simulink model "velocity_sin"  (R2015b)
settings: Solver=FixedStepDiscrete  StartTime=0.0  StopTime=inf  RelTol=1e-3
undefined symbols (not defined in the file or in its folder): DiscIntNeverNeededParam, Down, GPTRIP1SEL, GPTRIP2SEL, PWM_Counter_Period, TZ1, TZ2, Up
libraries: c280xlib x3, simulink x3, c2806xlib x2, dspsigops x2, c2802xlib x1
settings Model: ExtModeTrigDuration=10  Creator=Kalman  LastModifiedBy=ata.otaran
settings DataIOCC: SaveFormat=Array
settings OptimizationCC: OptimizeModelRefInitCode=on  LifeSpan=Inf  MaxStackSize=512
settings HardwareCC: ProdBitPerChar=16  ProdBitPerInt=16  ProdBitPerPointer=16  ProdLargestAtomicInteger=Integer  ProdLargestAtomicFloat=None  ProdWordSize=16  ProdLongLongMode=on  ProdHWDeviceType=Texas Instruments->C2000
settings RTWCC: SystemTargetFile=ert.tlc  TemplateMakefile=ert_default_tmf  Description=Embedded Coder  Toolchain=Texas Instruments Code Composer Studio v5 (C2000)
settings CodeAppCC: IgnoreCustomStorageClasses=off
settings ERTTargetCC: CodeReplacementLibrary=TI C28x
settings ConfigComp: CovModelRefEnable=Off

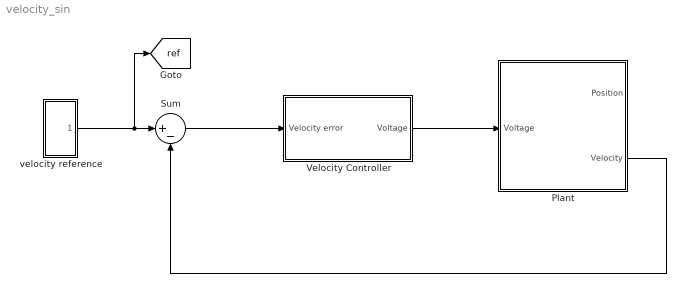
== system velocity_sin ==
  Plant : Subsystem
  Sum : Sum  Inputs=|+-
  Velocity Controller : Subsystem
  velocity reference : Subsystem
  tag scope: ref=global
  wires:
  Sum/1 -> Velocity Controller/1("Velocity error ")
  velocity reference/1(vref) -> [ref], Sum/1
  Plant/2(Velocity) -> Sum/2
  Velocity Controller/1(Voltage) -> Plant/1(Voltage)

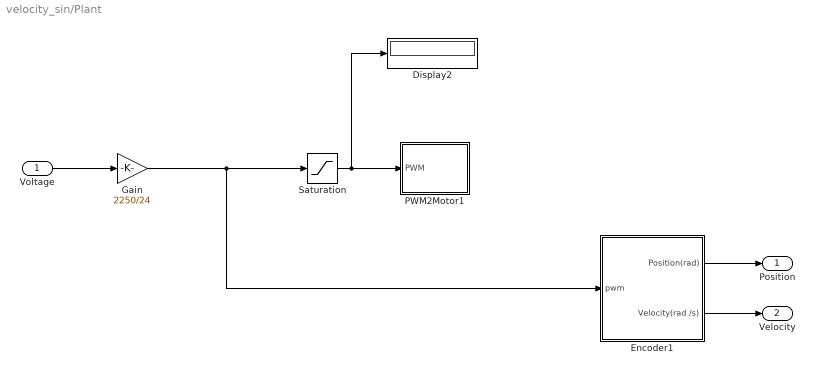
== system velocity_sin/Plant ==
  Voltage : Inport
  Display2 : Display
  Encoder1 : Subsystem
  Gain : Gain  Gain=2250/24
  PWM2Motor1 : Subsystem
  Saturation : Saturate  UpperLimit=2250  LowerLimit=-2250
  Position : Outport
  Velocity : Outport  Port=2
  wires:
  Encoder1/1("Position(rad) ") -> Position/1
  Encoder1/2(Velocity(rad /s)) -> Velocity/1
  Saturation/1 -> PWM2Motor1/1(PWM), Display2/1
  Gain/1 -> Saturation/1, Encoder1/1(pwm)
  Voltage/1 -> Gain/1

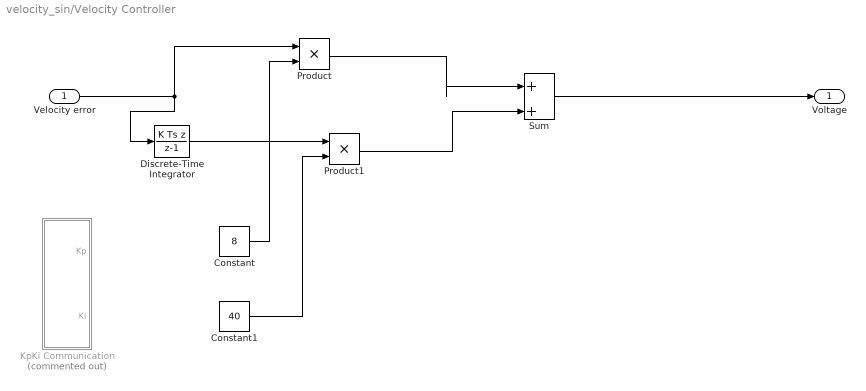
== system velocity_sin/Velocity Controller ==
  "Velocity error " : Inport
  Constant : Constant  Value=8
  Constant1 : Constant  Value=40
  Discrete-Time Integrator : DiscreteIntegrator  IntegratorMethod=Integration: Backward Euler  InitialConditionSetting=State (most efficient)  SampleTime=-1  ICPrevOutput=DiscIntNeverNeededParam  ICPrevScaledInput=DiscIntNeverNeededParam
  KpKi Communication : Subsystem  Commented=on
  Product : Product
  Product1 : Product
  Sum : Sum  Inputs=|++
  Voltage : Outport
  wires:
  "Velocity error "/1 -> Product/1, Discrete-Time Integrator/1
  Product/1 -> Sum/1
  Product1/1 -> Sum/2
  Discrete-Time Integrator/1 -> Product1/1
  Sum/1 -> Voltage/1
  Constant/1 -> Product/2
  Constant1/1 -> Product1/2

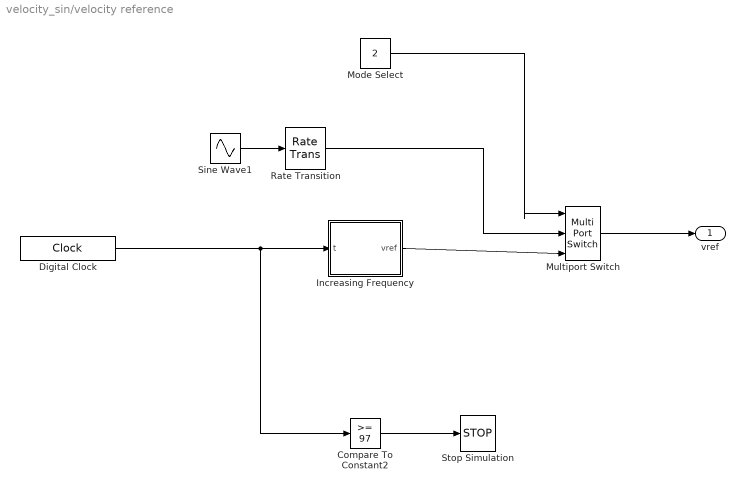
== system velocity_sin/velocity reference ==
  Compare To Constant2 : simulink/Logic and Bit Operations/Compare To Constant  relop=>=  const=97  OutDataTypeStr=boolean
  Digital Clock : DigitalClock  SampleTime=0.0001
  Increasing Frequency : Subsystem
  Mode Select : Constant  Value=2
  Multiport Switch : MultiPortSwitch  Inputs=2
  Rate Transition : RateTransition
  Sine Wave1 : Sin  Amplitude=5  Frequency=2*pi
  Stop Simulation : Stop
  vref : Outport
  wires:
  Sine Wave1/1 -> Rate Transition/1
  Digital Clock/1 -> Compare To Constant2/1, Increasing Frequency/1(t)
  Compare To Constant2/1 -> Stop Simulation/1
  Increasing Frequency/1(vref) -> Multiport Switch/3
  Rate Transition/1 -> Multiport Switch/2
  Multiport Switch/1 -> vref/1
  Mode Select/1 -> Multiport Switch/1

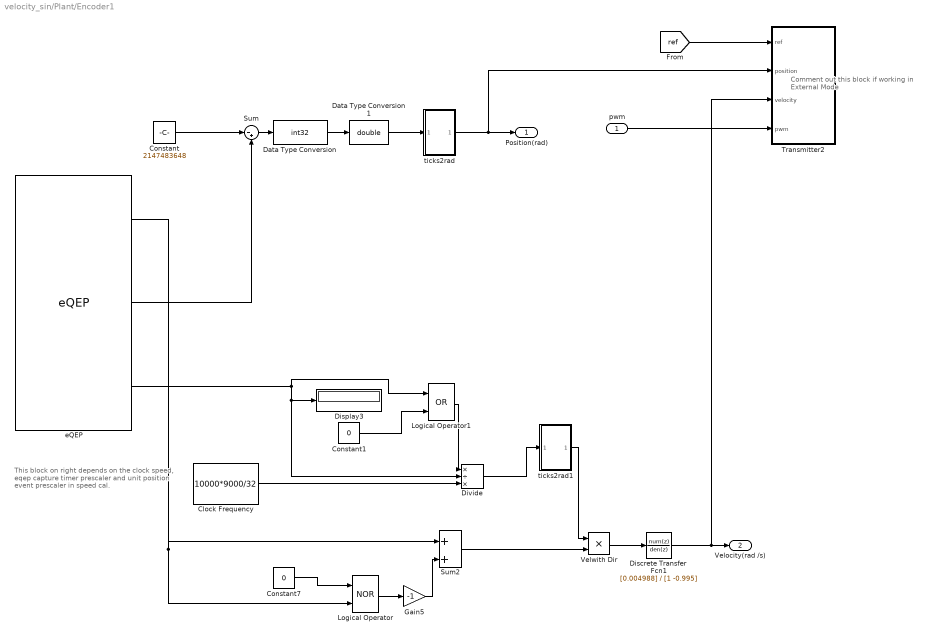
== system velocity_sin/Plant/Encoder1 ==
  note: Comment out this block if
      | working in External Mode
  note: This block on right depends on the clock speed, eqep capture timer prescaler and
      | unit position event prescaler in speed cal.
  pwm : Inport
  Clock Frequency : Constant  Value=10000*9000/32
  Constant : Constant  Value=2147483648  OutDataTypeStr=uint32
  Constant1 : Constant  Value=0
  Constant7 : Constant  Value=0
  Data Type Conversion : DataTypeConversion  OutDataTypeStr=int32
  Data Type Conversion1 : DataTypeConversion  OutDataTypeStr=double
  Discrete Transfer Fcn1 : DiscreteTransferFcn  Numerator=[0.004988]  Denominator=[1 -0.995]
  Display3 : Display
  Divide : Product  Inputs=*/*
  Gain5 : Gain  Gain=-1
  Logical Operator : Logic  Operator=NOR  AllPortsSameDT=off  OutDataTypeStr=boolean
  Logical Operator1 : Logic  Operator=OR  AllPortsSameDT=off  OutDataTypeStr=boolean
  Sum : Sum  Inputs=|-+
  Sum2 : Sum  Inputs=|++
  Transmitter2 : Subsystem
  "Velwith Dir " : Product
  eQEP : c280xlib/eQEP  useModule=eQEP1  pcInputmode=Quadrature-count  externalClockrate=2x resolution: Count the rising/falling edge  swapPolarityselection=Clockwise  qdfOutputport=on  qapPolarityselection=off  qbpPolarityselection=off  qipPolarityselection=off  qspPolarityselection=off  igatePolarityselection=off  sampleTime=0.0001  pcOutputport=on  pcMaximumvalue=4294967295  indexInitializationcheck=off  indexInitializationevent=Rising edge  strobeInitializationcheck=off  strobeInitializationevent=Rising edge  softwareInitializationcheck=on  softwareInitializationsource=Set to init value at start up  softwareInitializationmode=on  pcInitialvalue=2147483648  pcResetmode=Reset on an index event  ieloutputport=off  indexEventlatch=Rising edge  seloutputport=off  strobeEventlatch=Rising edge  pcefOutputport=off  enableEqepcapture=on  qctmrOutputport=off  qcprdOutputport=on  captureTimerprescaler=128  upEventprescaler=4  overflowErrorflag=off  directionErrorflag=off  captureTimerposition=On position counter read  unitTimerperiod=1000000000  captureTimerlatch=off  capturePeriodlatch=off  positionCounterlatch=off  soenPolarityselection=off  spselPolarityselection=Index pin is used for sync output  compareValuesource=Specify via dialog  shadowMode=Load on QPOSCNT=0  compareValue=4294967295  syncOutputwidth=1  polaritySyncoutput=Active high  watchdogEnable=off  watchdogTimer=65535  outport1Datatype=auto  outport2Datatype=uint32  outport3Datatype=auto  outport4Datatype=auto  outport5Datatype=auto  outport6Datatype=auto  outport7Datatype=auto  outport8Datatype=auto  outport9Datatype=auto  outport10Datatype=auto  outport11Datatype=auto  outport12Datatype=auto  eqepinterrupt_pce=off  eqepinterrupt_qpe=off  eqepinterrupt_qdc=off  eqepinterrupt_wto=off  eqepinterrupt_pcu=off  eqepinterrupt_pco=off  eqepinterrupt_pcr=off  eqepinterrupt_pcm=off  eqepinterrupt_sel=off  eqepinterrupt_iel=off  eqepinterrupt_uto=off  pheOutputport=off  watchdogOutputport=off  outport13Datatype=auto  outport14Datatype=auto
  ticks2rad : Subsystem
  ticks2rad1 : Subsystem
  "Position(rad) " : Outport
  Velocity(rad /s) : Outport  Port=2
  wires:
  ticks2rad1/1(Out1) -> "Velwith Dir "/1
  Logical Operator1/1 -> Divide/1
  Clock Frequency/1 -> Divide/3
  Constant1/1 -> Logical Operator1/2
  Sum2/1 -> "Velwith Dir "/2
  Constant7/1 -> Logical Operator/1
  Logical Operator/1 -> Gain5/1
  Divide/1 -> ticks2rad1/1(In1)
  Gain5/1 -> Sum2/2
  eQEP/1 -> Logical Operator/2, Sum2/1
  eQEP/2 -> Sum/2
  Constant/1 -> Sum/1
  eQEP/3 -> Divide/2, Display3/1, Logical Operator1/1
  Data Type Conversion/1 -> Data Type Conversion1/1
  ticks2rad/1(Out1) -> Transmitter2/2(position), "Position(rad) "/1
  Sum/1 -> Data Type Conversion/1
  Data Type Conversion1/1 -> ticks2rad/1(In1)
  pwm/1 -> Transmitter2/4(pwm)
  "Velwith Dir "/1 -> Discrete Transfer Fcn1/1
  [ref] -> Transmitter2/1(ref)
  Discrete Transfer Fcn1/1 -> Transmitter2/3(velocity), Velocity(rad /s)/1

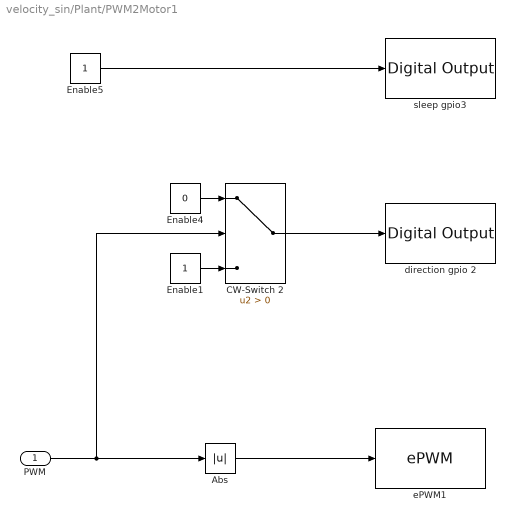
== system velocity_sin/Plant/PWM2Motor1 ==
  PWM : Inport
  Abs : Abs
  CW-Switch 2 : Switch  Criteria=u2 > Threshold
  Enable1 : Constant
  Enable4 : Constant  Value=0
  Enable5 : Constant
  direction gpio 2 : c2806xlib/Digital Output  GPIO_Number=GPIO0~GPIO7  GPIO_Bit0=off  GPIO_BIT0_Toggle=off  GPIO_Bit1=off  GPIO_BIT1_Toggle=off  GPIO_Bit2=on  GPIO_BIT2_Toggle=off  GPIO_Bit3=off  GPIO_BIT3_Toggle=off  GPIO_Bit4=off  GPIO_BIT4_Toggle=off  GPIO_Bit5=off  GPIO_BIT5_Toggle=off  GPIO_Bit6=off  GPIO_BIT6_Toggle=off  GPIO_Bit7=off  GPIO_BIT7_Toggle=off
  ePWM1 : c2802xlib/ePWM  useModule=ePWM1  ePWMxLINKTBPRD=Not Linked  periodUnits=Clock cycles  timerSource=Specify via dialog  timerPeriod_clk=PWM_Counter_Period+1  timerPeriod_sec=0.0001  tbshadow=Counter equals to zero  countingMode=Up-Down  phaseActiveEnable=Disable  phaseDirection=Count down after sync  phaseActive=0  synchronizationEnable=off  dcaevt1Sync=off  dcbevt1Sync=off  synchronizationOption=Disable  clockPrescale=1  HSclockPrescale=1  enswap=off  ePWMxAStatus=on  ePWMxAactionLogic1=Do nothing  ePWMxAactionLogic2=Do nothing  ePWMxAactionLogic3=Clear  ePWMxAactionLogic4=Set  ePWMxAactionLogic5=Do nothing  ePWMxAactionLogic6=Do nothing  ePWMxALoadMode=Load on counter equals to zero (CTR=Zero)  ePWMxACSFenable=off  ePWMxACSFvalue=Forcing disable  ePWMxASFreload=Zero  ePWMxBStatus=off  ePWMxBactionLogic1=Set  ePWMxBactionLogic2=Clear  ePWMxBactionLogic3=Do nothing  ePWMxBactionLogic4=Do nothing  ePWMxBactionLogic5=Clear  ePWMxBactionLogic6=Set  ePWMxBLoadMode=Load on counter equals to zero (CTR=Zero)  ePWMxBCSFenable=off  ePWMxBCSFvalue=Forcing disable  ePWMxBSFreload=Zero  ePWNxBOutWay=off  ePWMxLINKCMPA=Not Linked  CMPAUnits=Clock cycles  CMPASource=Input port  CMPAValue_per=50  CMPAValue_clk=PWM_Counter_Period/2+1  enCMPAshadow=Counter equals to zero  ePWMxLINKCMPB=Not Linked  CMPBUnits=Clock cycles  CMPBSource=Specify via dialog  CMPBValue_per=50  CMPBValue_clk=PWM_Counter_Period/2+1  enCMPBshadow=Counter equals to zero  ePWMxLINKCMPC=Not Linked  CMPCUnits=Clock cycles  CMPCSource=Specify via dialog  CMPCValue_per=50  CMPCValue_clk=32000  enCMPCshadow=Counter equals to zero  ePWMxLINKCMPD=Not Linked  CMPDUnits=Clock cycles  CMPDSource=Specify via dialog  CMPDValue_per=50  CMPDValue_clk=32000  enCMPDshadow=Counter equals to zero  enableDBePWMxA=off  enableDBePWMxB=off  enhalfcycle=off  DBpolarity=Active high (AH)  DBedgeDelay=Positive  DBSource_ePWMxA=ePWMxA  DBSource_ePWMxB=ePWMxA  DBperiodSource=Specify via dialog  REDperiod=0  FEDperiod=0  adcstartModuleA=off  adcrequestEventA=First event  adcstartEventA=Digital Compare Module A Event 1 start of conversion (DCAEVT1.soc)  adcstartEventA_type2=Digital Compare Module A Event 1 start of conversion (DCAEVT1.soc)  adcstartModuleB=off  adcrequestEventB=First event  adcstartEventB=Counter equals to zero (CTR=Zero)  adcstartEventB_type2=Counter equals to zero (CTR=Zero)  intEn=off  intPrd=First event  intSel=Counter equals to zero (CTR=Zero)  intSel_type2=Counter equals to zero (CTR=Zero)  hrpe=off  enHRPWM=off  HRPWM_LoadMode=Counter equals to period (CTR=PRD)  HRPWM_CTLMode=Duty or Period control mode  HRPWM_EDGMode=Both edge  hrpeb=off  enHRPWMB=off  HRPWM_LoadModeB=Counter equals to zero (CTR=ZERO)  HRPWM_CTLModeB=Duty or Period control mode  HRPWM_EDGModeB=Both edge  enSFO=on  enautoconv=on  chopperEnable=off  chopperFrequency=1  chopperFirstwidth=1  chopperDuty=12.5%  tripZonesource=Specify via dialog  tzselOSHT1=off  tzselOSHT2=off  tzselOSHT3=off  tzselOSHDCAEV1=off  tzselOSHDCBEV1=off  tzselCBC1=off  tzselCBC2=off  tzselCBC3=off  tzselCBCDCAEV2=off  tzselCBCDCBEV2=off  tzselOSHT4=off  tzselOSHT5=off  tzselOSHT6=off  tzselCBC4=off  tzselCBC5=off  tzselCBC6=off  enTzOstIntr=off  enTzCbcIntr=off  enTzDCAEVT1Intr=off  enTzDCAEVT2Intr=off  enTzDCBEVT1Intr=off  enTzDCBEVT2Intr=off  ePWMxAforced=No action  ePWMxBforced=No action  DCAEVT1forced=No action  DCBEVT1forced=No action  DCAEVT2forced=No action  DCBEVT2forced=No action  dcah=Trip Zone 1 input (TZ1)  dcal=Trip Zone 2 input (TZ2)  dcbh=Trip Zone 1 input (TZ1)  dcbl=Trip Zone 2 input (TZ2)  dcah_type2=GPTRIP1SEL/(TZ1)  dcal_type2=GPTRIP2SEL/(TZ2)  dcbh_type2=GPTRIP1SEL/(TZ1)  dcbl_type2=GPTRIP2SEL/(TZ2)  gendcaevt1=Event disabled  gendcaevt2=Event disabled  gendcbevt1=Event disabled  gendcbevt2=Event disabled  dcaevt1src=DCAEVT1 with sync  dcaevt2src=DCAEVT2 with sync  dcbevt1src=DCBEVT1 with sync  dcbevt2src=DCBEVT2 with sync  pulsesel=Counter equals to zero (CTR=Zero)  blankinv=off  blankoffset=0  blankwidth=0  evsrcsel=Filtered version of DCAEVT1 (DCAEVT1FILT)  encape=off  PwmType=C2000
  sleep gpio3 : c2806xlib/Digital Output  GPIO_Number=GPIO0~GPIO7  GPIO_Bit0=off  GPIO_BIT0_Toggle=off  GPIO_Bit1=off  GPIO_BIT1_Toggle=off  GPIO_Bit2=off  GPIO_BIT2_Toggle=off  GPIO_Bit3=on  GPIO_BIT3_Toggle=off  GPIO_Bit4=off  GPIO_BIT4_Toggle=off  GPIO_Bit5=off  GPIO_BIT5_Toggle=off  GPIO_Bit6=off  GPIO_BIT6_Toggle=off  GPIO_Bit7=off  GPIO_BIT7_Toggle=off
  wires:
  PWM/1 -> Abs/1, CW-Switch 2/2
  Enable1/1 -> CW-Switch 2/3
  Enable4/1 -> CW-Switch 2/1
  Enable5/1 -> sleep gpio3/1
  CW-Switch 2/1 -> direction gpio 2/1
  Abs/1 -> ePWM1/1

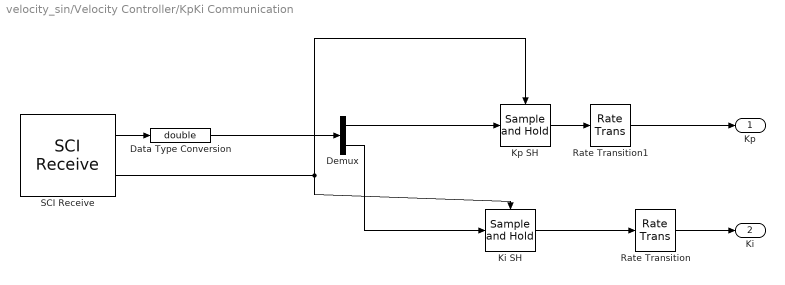
== system velocity_sin/Velocity Controller/KpKi Communication ==
  Data Type Conversion : DataTypeConversion  OutDataTypeStr=double
  Demux : Demux  Outputs=2
  Ki SH : dspsigops/Sample and Hold  trig=Rising edge  initCond=40  latchinput=off
  Kp SH : dspsigops/Sample and Hold  trig=Rising edge  initCond=8  latchinput=off
  Rate Transition : RateTransition
  Rate Transition1 : RateTransition
  SCI Receive : c280xlib/SCI Receive  sciModule=A  dataHead='S'  dataTail='E'  dataType=int32  dataDim=2  initValue=0  errOption=Output the last received value  errValue=0  sampleTime=0.05  outputStatus=on  postInterrupt=off  numFifo=1
  Kp : Outport
  Ki : Outport  Port=2
  wires:
  Demux/2 -> Ki SH/1
  SCI Receive/1 -> Data Type Conversion/1
  Rate Transition1/1 -> Kp/1
  Rate Transition/1 -> Ki/1
  SCI Receive/2 -> Kp SH/Trigger, Ki SH/Trigger
  Data Type Conversion/1 -> Demux/1
  Kp SH/1 -> Rate Transition1/1
  Demux/1 -> Kp SH/1
  Ki SH/1 -> Rate Transition/1

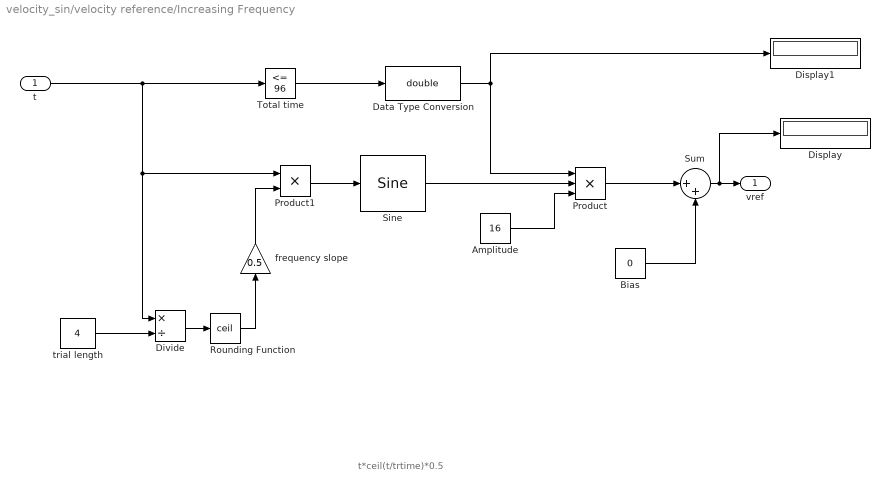
== system velocity_sin/velocity reference/Increasing Frequency ==
  note: t*ceil(t/trtime)*0.5
  t : Inport
  Amplitude : Constant  Value=16
  Bias : Constant  Value=0
  Data Type Conversion : DataTypeConversion  OutDataTypeStr=double  ConvertRealWorld=Stored Integer (SI)
  Display : Display
  Display1 : Display
  Divide : Product  Inputs=*/
  Product : Product  Inputs=3
  Product1 : Product
  Rounding Function : Rounding  Operator=ceil
  Sine : simulink/Lookup Tables/Sine  Formula=sin(2*pi*u)  NumDataPoints=(2^5)+1  OutputWordLength=16  InternalRulePriority=Speed
  Sum : Sum  Inputs=|++
  Total time : simulink/Logic and Bit Operations/Compare To Constant  relop=<=  const=96  OutDataTypeStr=boolean
  frequency slope : Gain  Gain=0.5
  trial length : Constant  Value=4  SampleTime=-1
  vref : Outport
  wires:
  Rounding Function/1 -> frequency slope/1
  Product1/1 -> Sine/1
  Data Type Conversion/1 -> Product/1, Display1/1
  trial length/1 -> Divide/2
  Total time/1 -> Data Type Conversion/1
  Sum/1 -> vref/1, Display/1
  t/1 -> Total time/1, Divide/1, Product1/1
  Divide/1 -> Rounding Function/1
  Sine/1 -> Product/2
  Amplitude/1 -> Product/3
  frequency slope/1 -> Product1/2
  Product/1 -> Sum/1
  Bias/1 -> Sum/2

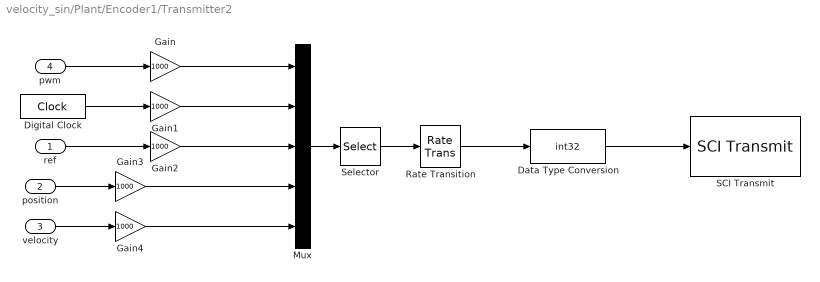
== system velocity_sin/Plant/Encoder1/Transmitter2 ==
  ref : Inport
  position : Inport  Port=2
  velocity : Inport  Port=3
  pwm : Inport  Port=4
  Data Type Conversion : DataTypeConversion  OutDataTypeStr=int32  ConvertRealWorld=Stored Integer (SI)
  Digital Clock : DigitalClock  SampleTime=0.0001
  Gain{,1..4} (5 alike) : Gain  Gain=1000
  Mux : Mux  Inputs=5
  Rate Transition : RateTransition  Integrity=off  OutPortSampleTime=0.02
  SCI Transmit : c280xlib/SCI Transmit  sciModule=A  dataHead='S'  dataTail='E'  postInterrupt=on  numFifo=3
  Selector : Selector  InputPortWidth=5  IndexOptions=Index vector (dialog)  Indices=[2 5]  OutputSizes=1
  wires:
  Rate Transition/1 -> Data Type Conversion/1
  Data Type Conversion/1 -> SCI Transmit/1
  velocity/1 -> Gain4/1
  Digital Clock/1 -> Gain1/1
  Gain/1 -> Mux/1
  pwm/1 -> Gain/1
  ref/1 -> Gain2/1
  Mux/1 -> Selector/1
  Gain1/1 -> Mux/2
  Selector/1 -> Rate Transition/1
  position/1 -> Gain3/1
  Gain2/1 -> Mux/3
  Gain3/1 -> Mux/4
  Gain4/1 -> Mux/5

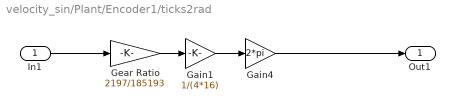
== system velocity_sin/Plant/Encoder1/ticks2rad ==
  In1 : Inport
  Gain1 : Gain  Gain=1/(4*16)
  Gain4 : Gain  Gain=2*pi
  Gear Ratio : Gain  Gain=2197/185193
  Out1 : Outport
  wires:
  Gain1/1 -> Gain4/1
  Gear Ratio/1 -> Gain1/1
  In1/1 -> Gear Ratio/1
  Gain4/1 -> Out1/1

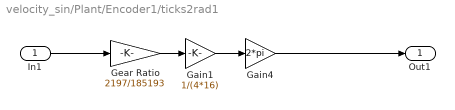
== system velocity_sin/Plant/Encoder1/ticks2rad1 ==
  In1 : Inport
  Gain1 : Gain  Gain=1/(4*16)
  Gain4 : Gain  Gain=2*pi
  Gear Ratio : Gain  Gain=2197/185193
  Out1 : Outport
  wires:
  Gain1/1 -> Gain4/1
  Gear Ratio/1 -> Gain1/1
  In1/1 -> Gear Ratio/1
  Gain4/1 -> Out1/1
